simulink subsystem "dq2dp"  (R2023a)
settings: Solver=VariableStepAuto  StartTime=0.0  StopTime=10.0  RelTol=1e-3
settings Model: Creator=lukasz  LastModifiedBy=lukasz

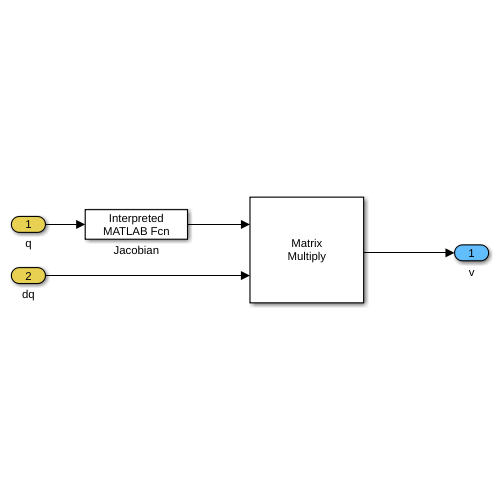
[thumbnail: Simulink's stored preview of the top-level diagram]
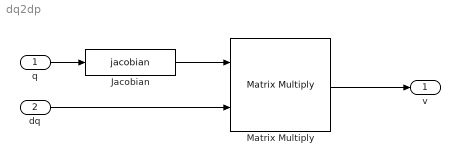
== system dq2dp ==
  q : Inport
  dq : Inport  Port=2
  Jacobian : MATLABFcn  MATLABFcn=jacobian  Output1D=off
  Matrix Multiply : Product  Multiplication=Matrix(*)
  v : Outport
  wires:
  q/1 -> Jacobian/1
  dq/1 -> Matrix Multiply/2
  Matrix Multiply/1 -> v/1
  Jacobian/1 -> Matrix Multiply/1
